simulink model "Einmassensystem"  (R2022b)
settings: Solver=ode45  StartTime=0.0  StopTime=5  RelTol=1e-6  EnableMultiTasking=on
values from neighbouring files (symbols this model uses):
  A_a = [0 1 0 ... (first row only)    [Parameter_kalmanfilter.m]
  B_a = [0; 0; 1/T_EM]    [Parameter_kalmanfilter.m]
  Bz_a = [0; -1/J; 0]    [Parameter_kalmanfilter.m]
  Ce_a = [1 0 0]    [Parameter_kalmanfilter.m]
  Ce_b = [Ce_a 0]    [Parameter_kalmanfilter.m]
  H_a = [ (1/J)*(T^2/2 - T_EM*T + T_EM^2*(1-alpha)) ... (first row only)    [Parameter_kalmanfilter.m]
  H_b = [ (1/J)*(T^2/2 - T_EM*T + T_EM^2*(1-alpha)) ... (first row only)    [Parameter_kalmanfilter.m]
  P_0_a = eye(3)    [Parameter_kalmanfilter.m]
  P_0_b = eye(4)    [Parameter_kalmanfilter.m]
  Phi_T_a = [ 1, T, (T_EM/J)*(T - T_EM*(1-alpha)) ... (first row only)    [Parameter_kalmanfilter.m]
  Phi_T_b = [ 1, T, (T_EM/J)*(T - T_EM*(1-alpha)),  -(T^2)/(2*J) ... (first row only)    [Parameter_kalmanfilter.m]
  Q_a = diag([10 10 10])    [Parameter_kalmanfilter.m]
  Q_b = diag([10 10 10 1000])    [Parameter_kalmanfilter.m]
  R_a = 1e-6    (= 1e-06)    [Parameter_kalmanfilter.m]
  R_b = 1e-6    (= 1e-06)    [Parameter_kalmanfilter.m]
  T = 1e-4    (= 0.0001)    [Parameter_kalmanfilter.m]
settings Model: Creator=masoud  LastModifiedBy=kraie
settings SolverCC: AlgebraicLoopSolver=TrustRegion
settings DataIOCC: ReturnWorkspaceOutputs=off
settings OptimizationCC: LifeSpan=inf
settings DebuggingCC: UnconnectedInputMsg=warning  UnconnectedOutputMsg=warning  UnconnectedLineMsg=warning  SFUnexpectedBacktrackingDiag=warning  SFNoUnconditionalDefaultTransitionDiag=warning  SFMachineParentedDataDiag=warning  ArithmeticOperatorsInVariantConditions=warning
settings ModelReferenceCC: EnableRefExpFcnMdlSchedulingChecks=on
settings SFSimCC: SimUseLocalCustomCode=off  CustomCodeUndefinedFunction=UseInterfaceOnly
settings RTWCC: RTWUseLocalCustomCode=off
settings CodeAppCC: StateflowObjectComments=on
settings GRTTargetCC: TargetLangStandard=C89/C90 (ANSI)
settings ConfigComp: CovMetricSettings=dw  CovSaveCumulativeToWorkspaceVar=on  CovSaveSingleToWorkspaceVar=on  CovExternalEMLEnable=off

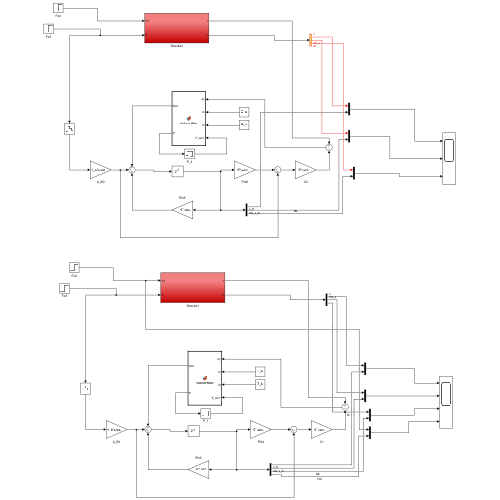
[thumbnail: Simulink's stored preview of the top-level diagram]
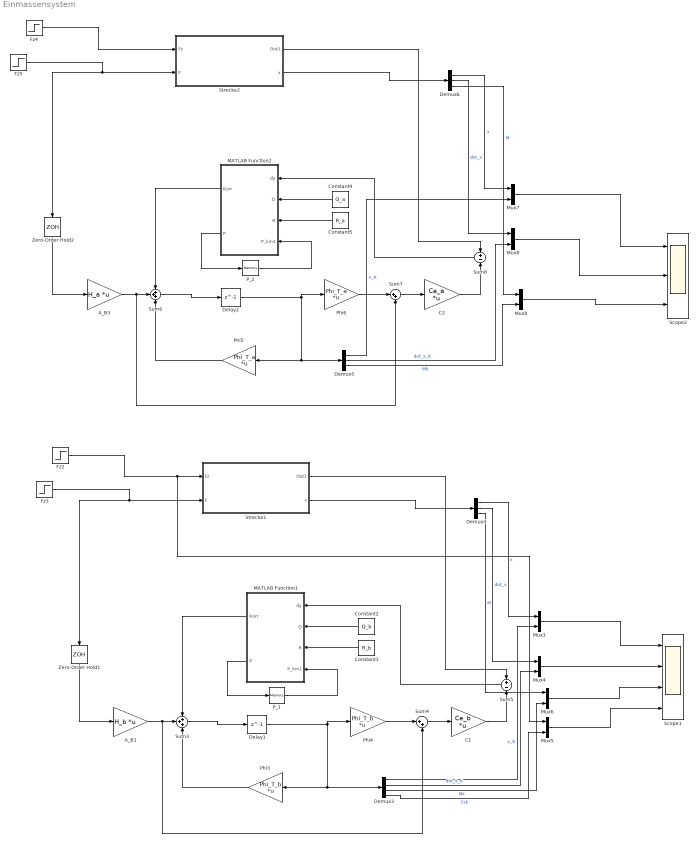
== system Einmassensystem ==
  A_B1 : Gain  Gain=H_b  Multiplication=Matrix(K*u) (u vector)
  A_B3 : Gain  Gain=H_a  Multiplication=Matrix(K*u) (u vector)
  C1 : Gain  Gain=Ce_b  Multiplication=Matrix(K*u) (u vector)
  C2 : Gain  Gain=Ce_a  Multiplication=Matrix(K*u) (u vector)
  Constant2 : Constant  Value=Q_b
  Constant3 : Constant  Value=R_b
  Constant4 : Constant  Value=Q_a
  Constant5 : Constant  Value=R_a
  Delay1 : Delay  DelayLength=1  InitialCondition=0  SampleTime=T
  Delay2 : Delay  DelayLength=1  InitialCondition=0  SampleTime=T
  Demux3 : Demux
  Demux4 : Demux  Outputs=3
  Demux5 : Demux  Outputs=3
  Demux6 : Demux  Outputs=3
  Fz2 : Step  SampleTime=0
  Fz3 : Step  Time=0.1  After=2  SampleTime=0
  Fz4 : Step  Time=0  After=0  SampleTime=0
  Fz5 : Step  Time=0.1  After=2  SampleTime=0
  MATLAB Function1 : MATLAB Function  TreatAsAtomicUnit=on
  MATLAB Function2 : MATLAB Function  TreatAsAtomicUnit=on
  Mux{3..9} (7 alike) : Mux  Inputs=2
  P_1 : Memory  InitialCondition=P_0_b
  P_2 : Memory  InitialCondition=P_0_a
  Phi3 : Gain  Gain=Phi_T_b  Multiplication=Matrix(K*u) (u vector)
  Phi4 : Gain  Gain=Phi_T_b  Multiplication=Matrix(K*u) (u vector)
  Phi5 : Gain  Gain=Phi_T_a  Multiplication=Matrix(K*u) (u vector)
  Phi6 : Gain  Gain=Phi_T_a  Multiplication=Matrix(K*u) (u vector)
  Scope1 : Scope  NumInputPorts=4
  Scope2 : Scope  NumInputPorts=3
  Strecke1 : Subsystem
  Strecke2 : Subsystem
  Sum3 : Sum  Inputs=+++
  Sum4 : Sum  Inputs=|++
  Sum5 : Sum  Inputs=+-
  Sum6 : Sum  Inputs=+++
  Sum7 : Sum  Inputs=|++
  Sum8 : Sum  Inputs=+-
  Zero-Order Hold1 : ZeroOrderHold  SampleTime=T
  Zero-Order Hold2 : ZeroOrderHold  SampleTime=T
  wires:
  Demux4/2 -> Mux4/1  "dot_x"
  Zero-Order Hold1/1 -> A_B1/1
  Sum4/1 -> C1/1
  Mux5/1 -> Scope1/4
  A_B1/1 -> Sum4/2, Sum3/2
  Demux3/3 -> Mux6/2  "Mk"
  Demux4/1 -> Mux3/1  "x"
  Strecke1/2(x) -> Demux4/1
  Demux3/1 -> Mux3/2  "x_K"
  Sum3/1 -> Delay1/1
  Fz3/1 -> Zero-Order Hold1/1, Strecke1/2(F)
  MATLAB Function1/2(P) -> P_1/1
  P_1/1 -> MATLAB Function1/4(P_km1)
  Demux3/2 -> Mux4/2  "dot_x_K"
  Fz2/1 -> Mux5/1, Strecke1/1(Fz)
  Phi3/1 -> Sum3/3
  Constant2/1 -> MATLAB Function1/2(Q)
  Phi4/1 -> Sum4/1
  MATLAB Function1/1(Korr) -> Sum3/1
  Delay1/1 -> Phi4/1, Phi3/1, Demux3/1
  Constant3/1 -> MATLAB Function1/3(R)
  Sum5/1 -> MATLAB Function1/1(dy)
  C1/1 -> Sum5/2
  Strecke1/1(Out1) -> Sum5/1
  Mux3/1 -> Scope1/1
  Mux4/1 -> Scope1/2
  Demux3/4 -> Mux5/2  "Fzk"
  Demux4/3 -> Mux6/1  "M"
  Mux6/1 -> Scope1/3
  Mux8/1 -> Scope2/2
  Mux7/1 -> Scope2/1
  Demux5/3 -> Mux9/2  "Mk"
  Phi6/1 -> Sum7/1
  Mux9/1 -> Scope2/3
  Sum8/1 -> MATLAB Function2/1(dy)
  MATLAB Function2/2(P) -> P_2/1
  Demux5/2 -> Mux8/2  "dot_x_K"
  MATLAB Function2/1(Korr) -> Sum6/1
  Constant4/1 -> MATLAB Function2/2(Q)
  Constant5/1 -> MATLAB Function2/3(R)
  Delay2/1 -> Phi6/1, Phi5/1, Demux5/1
  C2/1 -> Sum8/2
  Strecke2/2(x) -> Demux6/1
  Phi5/1 -> Sum6/3
  Sum7/1 -> C2/1
  A_B3/1 -> Sum7/2, Sum6/2
  Demux6/1 -> Mux7/1  "x"
  Fz5/1 -> Zero-Order Hold2/1, Strecke2/2(F)
  Fz4/1 -> Strecke2/1(Fz)
  P_2/1 -> MATLAB Function2/4(P_km1)
  Sum6/1 -> Delay2/1
  Zero-Order Hold2/1 -> A_B3/1
  Strecke2/1(Out1) -> Sum8/1
  Demux5/1 -> Mux7/2  "x_K"
  Demux6/3 -> Mux9/1  "M"
  Demux6/2 -> Mux8/1  "dot_x"

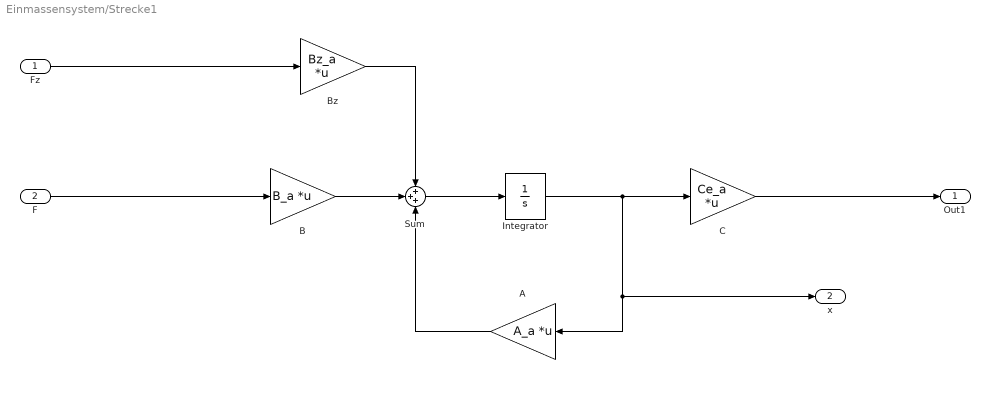
== system Einmassensystem/Strecke1 ==
  Fz : Inport
  F : Inport  Port=2
  A : Gain  Gain=A_a  Multiplication=Matrix(K*u) (u vector)
  B : Gain  Gain=B_a  Multiplication=Matrix(K*u) (u vector)
  Bz : Gain  Gain=Bz_a  Multiplication=Matrix(K*u) (u vector)
  C : Gain  Gain=Ce_a  Multiplication=Matrix(K*u) (u vector)
  Integrator : Integrator
  Sum : Sum  Inputs=+++
  Out1 : Outport
  x : Outport  Port=2
  wires:
  B/1 -> Sum/2
  A/1 -> Sum/3
  C/1 -> Out1/1
  F/1 -> B/1
  Sum/1 -> Integrator/1
  Integrator/1 -> x/1, A/1, C/1
  Bz/1 -> Sum/1
  Fz/1 -> Bz/1

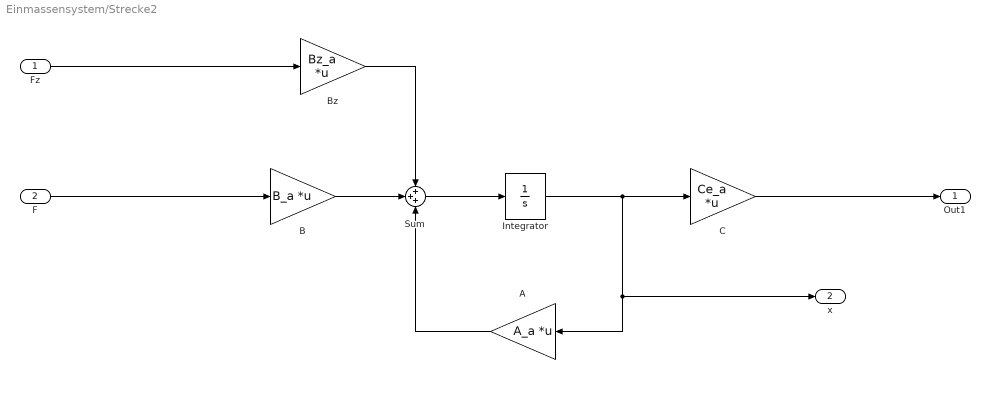
== system Einmassensystem/Strecke2 ==
  Fz : Inport
  F : Inport  Port=2
  A : Gain  Gain=A_a  Multiplication=Matrix(K*u) (u vector)
  B : Gain  Gain=B_a  Multiplication=Matrix(K*u) (u vector)
  Bz : Gain  Gain=Bz_a  Multiplication=Matrix(K*u) (u vector)
  C : Gain  Gain=Ce_a  Multiplication=Matrix(K*u) (u vector)
  Integrator : Integrator
  Sum : Sum  Inputs=+++
  Out1 : Outport
  x : Outport  Port=2
  wires:
  B/1 -> Sum/2
  A/1 -> Sum/3
  C/1 -> Out1/1
  F/1 -> B/1
  Sum/1 -> Integrator/1
  Integrator/1 -> x/1, A/1, C/1
  Bz/1 -> Sum/1
  Fz/1 -> Bz/1

== matlab function Einmassensystem/MATLAB Function1 ==
  data: dy input; Korr output; Q input; R input; Phi_T_b parameter; Ce_b parameter; P output; P_km1 input
function [Korr,P] = Kalmanfilter(dy,Q,R,Phi_T_b,Ce_b,P_km1)

Ps = Phi_T_b*P_km1*Phi_T_b'+Q;
K  = Ps*Ce_b'*(1/(Ce_b*Ps*Ce_b'+R));
P  = (eye(4)-K*Ce_b)*Ps*(eye(4)-K*Ce_b)'+K*R*K';

Korr = K*dy;
end

== matlab function Einmassensystem/MATLAB Function2 ==
  data: dy input; Korr output; Q input; R input; Phi_T_a parameter; Ce_a parameter; P output; P_km1 input
function [Korr,P] = Kalmanfilter(dy,Q,R,Phi_T_a,Ce_a,P_km1)

Ps = Phi_T_a*P_km1*Phi_T_a'+Q;
K  = Ps*Ce_a'*(1/(Ce_a*Ps*Ce_a'+R));
P  = (eye(3)-K*Ce_a)*Ps*(eye(3)-K*Ce_a)'+K*R*K';

Korr = K*dy;
end
